simulink subsystem "WindGFMCap23a"  (R2023a)
settings: Solver=VariableStepAuto  StartTime=0.0  StopTime=10.0  RelTol=1e-3
model mask{x_vir1=0, r_vir1=0, Imax1=0, Kt=0, Kj=0, Kd=0, frequency1=0, V_ref=0, Kq=0, Q_ref=0, Kpd_mpp=0, Kid_mpp=0, Kpq_mpp=0, Kiq_mpp=0, p=0, psim=0, Ld=0, Lq=0, Rs=0, Radius=0, pitch=0, cp=0, TSR=0, airDensity=0, wt=0, rt=0, Inertia=0}
  mask prompts: x_vir1 "Virtual reactance"; r_vir1 "Virtual resistance"; Imax1 "Current limit saturation"; Kt "Tracking Cofficient"; Kj "Inertia Cofficient"; Kd "Damping Cofficient"; frequency1 "Frequency reference"; V_ref "Voltage Reference (PU)"; Kq "Reactive Power Droop"; Q_ref "Reactive Power Reference"; Kpd_mpp "D-axis Proportional Gain"; Kid_mpp "D-axis Integral Gain"; Kpq_mpp "Q-axis Proportional Gain"; Kiq_mpp "Q-axis Integral Gain"; p "Number of Pole Pairs"; psim "PMSM Flux linkage (Wb)"; Ld "Stator D-axis inductance (H)"; Lq "Stator Q-axis inductance (H)"; Rs "Stator Resistance (Ohms)"; Radius "Turbine Radious"; pitch "Turbine Pitch Angle Vector"; cp "Power Cofficient"; TSR "Tip Speed Ratio"; airDensity "Air Density"; wt "Wind Velocity Threshold"; rt "Rotational Velocity Threshold"; Inertia "Turbine Inertia"
undefined symbols (not defined in the file): alpha, base, DiscIntNeverNeededParam, gGFMTfz, mpptPower, mpptWindSpeed, Ts, windController, windInverter, windTurbine
libraries: nesl_utility x15, ee_lib x11, fl_lib x8, eeTransforms x5, slpidlib x4, eeGeneralControl x2, simulink x2, simulink_extras x1, eePowerMeasurement x1, eePmsmCurrentController x1
(part 2 of 2)

== system WindGFMCap23a/Wind Turbine with Grid Forming /Machine-side Converter Control/Power Controller/MPPT Control ==
  windSpeed : Inport
  Enable : EnablePort  StatesWhenEnabling=reset
  MW to W : Gain  Gain=1e6
  mpptActivePowerDemand : Lookup_n-D  NumberOfTableDimensions=1  BreakpointsForDimension1=mpptWindSpeed  Table=mpptPower*4  InternalRulePriority=Speed  RndMeth=Simplest
  activePowerDemand : Outport
  wires:
  MW to W/1 -> activePowerDemand/1
  windSpeed/1 -> mpptActivePowerDemand/1
  mpptActivePowerDemand/1 -> MW to W/1
